simulink model "cantoni_combined_matrices_3pools_split"  (R2019b)
settings: Solver=FixedStepDiscrete  StartTime=0.0  StopTime=50  FixedStep=h  RelTol=1e-3
values from neighbouring files (symbols this model uses):
  comb_contr = ss(Ac, Bc, Cc, Dc, h)    [cantoni_LMI.m]
  comb_plant_disc = c2d(comb_plant_cont,h,'zoh')    [cantoni_LMI.m]
  ddelay = [4 2 4 4 6]    [distributed_workspace.mat]
undefined symbols (not defined in the file or in its folder): Pd, Wd
settings Model: Creator=Jacob  LastModifiedBy=bas
settings SFSimCC: CustomCodeUndefinedFunction=UseInterfaceOnly

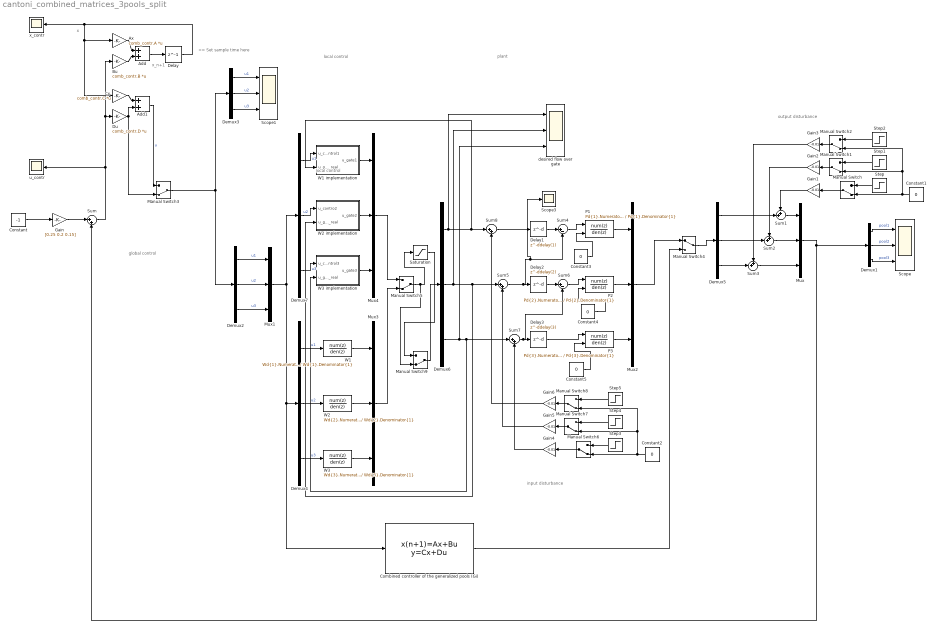
== system cantoni_combined_matrices_3pools_split ==
  note: input disturbance
  note: output disturbance
  note: local control
  note: <= Set sample time here
  note: plant
  note: local control
  note: global control
  note: x
  note: x_n+1
  Add : Sum
  Add1 : Sum
  Ax : Gain  Gain=comb_contr.A  Multiplication=Matrix(K*u)
  Bu : Gain  Gain=comb_contr.B  Multiplication=Matrix(K*u)
  Combined controller of the generalized pools (Gi) : DiscreteStateSpace  A=comb_plant_disc.A  B=comb_plant_disc.B  C=comb_plant_disc.C  D=comb_plant_disc.D  SampleTime=-1
  Constant : Constant  Value=-1
  Constant{1..2,4..5} (4 alike) : Constant  Value=0
  Constant3 : Constant  Value=0  SampleTime=-1
  Cx : Gain  Gain=comb_contr.C  Multiplication=Matrix(K*u)
  Delay : Delay  DelayLength=1  InitialCondition=[0;0;0;0;0;0;0;0;0;0;0;0;0;0;0]
  Delay1 : Delay  DelayLength=ddelay(1)
  Delay2 : Delay  DelayLength=ddelay(2)
  Delay3 : Delay  DelayLength=ddelay(3)
  Demux{1..7} (7 alike) : Demux  Outputs=3
  Du : Gain  Gain=comb_contr.D  Multiplication=Matrix(K*u)
  Gain : Gain  Gain=[0.25 0.2 0.15]
  Gain{1..6} (6 alike) : Gain  Gain=-0.01
  Manual Switch{,1..3,5..9} (9 alike) : ManualSwitch  CurrentSetting=0
  Manual Switch4 : ManualSwitch
  Mux{,1..4} (5 alike) : Mux  Inputs=3
  P1 : DiscreteTransferFcn  Numerator=Pd{1}.Numerator{1}  Denominator=Pd{1}.Denominator{1}  InitialStatesSource=Input port
      settings: InputPortMap=u0,p5
  P2 : DiscreteTransferFcn  Numerator=Pd{2}.Numerator{1}  Denominator=Pd{2}.Denominator{1}  InitialStatesSource=Input port
      settings: InputPortMap=u0,p5
  P3 : DiscreteTransferFcn  Numerator=Pd{3}.Numerator{1}  Denominator=Pd{3}.Denominator{1}  InitialStatesSource=Input port
      settings: InputPortMap=u0,p5
  Saturation : Saturate  UpperLimit=0.005  LowerLimit=-0.0001
  Scope : Scope  NumInputPorts=3
  Scope1 : Scope  NumInputPorts=3
  Scope3 : Scope
  Step{,1..5} (6 alike) : Step  Time=50  SampleTime=0
  Sum{,5,7..8} (4 alike) : Sum  Inputs=|++
  Sum1 : Sum  Inputs=++|
  Sum2 : Sum  Inputs=++|
  Sum3 : Sum  Inputs=++|
  Sum4 : Sum  Inputs=|+-
  Sum6 : Sum  Inputs=|+-
  W1 : DiscreteTransferFcn  Numerator=Wd{1}.Numerator{1}  Denominator=Wd{1}.Denominator{1}
  W1 implementation : Subsystem
  W2 : DiscreteTransferFcn  Numerator=Wd{2}.Numerator{1}  Denominator=Wd{2}.Denominator{1}
  W2 implementation : Subsystem
  W3 : DiscreteTransferFcn  Numerator=Wd{3}.Numerator{1}  Denominator=Wd{3}.Denominator{1}
  W3 implementation : Subsystem
  desired flow over gate : Scope  NumInputPorts=3
  u_contr : Scope
  x_contr : Scope
  wires:
  Sum/1 -> Du/1, Bu/1, u_contr/1
  Constant/1 -> Gain/1
  Gain/1 -> Sum/1
  Mux/1 -> Demux1/1, Sum/2
  Demux1/1 -> Scope/1  "pool1"
  Demux1/2 -> Scope/2  "pool2"
  Demux1/3 -> Scope/3  "pool3"
  Step/1 -> Manual Switch/1
  Sum1/1 -> Mux/1
  Sum2/1 -> Mux/2
  Gain2/1 -> Sum2/1
  Step1/1 -> Manual Switch1/1
  Gain1/1 -> Sum1/1
  Manual Switch/1 -> Gain1/1
  Constant1/1 -> Manual Switch1/2, Manual Switch2/2, Manual Switch/2
  Manual Switch1/1 -> Gain2/1
  Sum3/1 -> Mux/3
  Manual Switch2/1 -> Gain3/1
  Step2/1 -> Manual Switch2/1
  Gain3/1 -> Sum3/1
  Demux2/3 -> Mux1/3  "u3"
  Demux2/2 -> Mux1/2  "u2"
  Demux3/3 -> Scope1/3  "u3"
  Demux3/2 -> Scope1/2  "u2"
  Demux3/1 -> Scope1/1  "u1"
  Ax/1 -> Add/1
  Add/1 -> Delay/1
  Bu/1 -> Add/2
  Delay/1 -> x_contr/1, Cx/1, Ax/1
  Cx/1 -> Add1/1
  Du/1 -> Manual Switch3/2, Add1/2
  Add1/1 -> Manual Switch3/1  "u"
  Manual Switch3/1 -> Demux2/1, Demux3/1
  Demux2/1 -> Mux1/1  "u1"
  Demux5/1 -> Sum1/2
  Demux5/2 -> Sum2/2
  Demux5/3 -> Sum3/2
  Mux1/1 -> Combined controller of the generalized pools (Gi)/1, Demux4/1, Demux7/1
  Demux4/1 -> W1/1  "u1"
  Demux4/2 -> W2/1  "u2"
  Demux4/3 -> W3/1  "u3"
  Manual Switch4/1 -> Demux5/1
  P1/1 -> Mux2/1
  P2/1 -> Mux2/2
  P3/1 -> Mux2/3
  Mux2/1 -> Manual Switch4/1
  Combined controller of the generalized pools (Gi)/1 -> Manual Switch4/2
  Sum4/1 -> P1/1
  Sum6/1 -> P2/1
  Demux6/1 -> W1 implementation/2(u_gate1_real), Sum8/1, desired flow over gate/1
  Demux6/2 -> W2 implementation/2(u_gate2_real), Sum5/1, desired flow over gate/2
  Demux6/3 -> W3 implementation/2(u_gate3_real), Sum7/1, desired flow over gate/3
  Delay1/1 -> Sum4/1
  Delay2/1 -> Sum6/1
  Delay3/1 -> P3/1
  W1/1 -> Mux3/1
  W1 implementation/1(u_gate1) -> Mux4/1
  W2/1 -> Mux3/2
  W3/1 -> Mux3/3
  Mux3/1 -> Manual Switch5/2
  Demux7/1 -> W1 implementation/1(u_control1)  "u1"
  Mux4/1 -> Manual Switch5/1
  Demux7/2 -> W2 implementation/1(u_contro2)  "u2"
  W2 implementation/1(u_gate2) -> Mux4/2
  W3 implementation/1(u_gate3) -> Mux4/3
  Demux7/3 -> W3 implementation/1(u_control3)  "u3"
  Gain5/1 -> Sum5/2
  Gain4/1 -> Sum7/2
  Manual Switch8/1 -> Gain6/1
  Step5/1 -> Manual Switch8/1
  Gain6/1 -> Sum8/2
  Constant2/1 -> Manual Switch7/2, Manual Switch8/2, Manual Switch6/2
  Manual Switch7/1 -> Gain5/1
  Step3/1 -> Manual Switch6/1
  Manual Switch6/1 -> Gain4/1
  Step4/1 -> Manual Switch7/1
  Sum8/1 -> Delay1/1
  Sum5/1 -> Scope3/1, Sum4/2, Delay2/1
  Sum7/1 -> Sum6/2, Delay3/1
  Constant3/1 -> P1/2
  Saturation/1 -> Manual Switch9/1
  Constant4/1 -> P2/2
  Constant5/1 -> P3/2
  Manual Switch5/1 -> Manual Switch9/2, Saturation/1
  Manual Switch9/1 -> Demux6/1

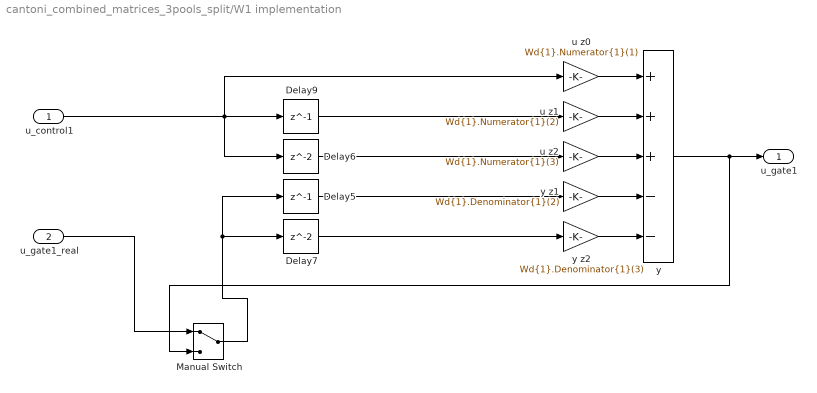
== system cantoni_combined_matrices_3pools_split/W1 implementation ==
  u_control1 : Inport
  u_gate1_real : Inport  Port=2
  Delay5 : Delay  DelayLength=1
  Delay6 : Delay
  Delay7 : Delay
  Delay9 : Delay  DelayLength=1
  Manual Switch : ManualSwitch
  u z0 : Gain  Gain=Wd{1}.Numerator{1}(1)
  u z1 : Gain  Gain=Wd{1}.Numerator{1}(2)
  u z2 : Gain  Gain=Wd{1}.Numerator{1}(3)
  y : Sum  Inputs=+++--
  y z1 : Gain  Gain=Wd{1}.Denominator{1}(2)
  y z2 : Gain  Gain=Wd{1}.Denominator{1}(3)
  u_gate1 : Outport
  wires:
  y z2/1 -> y/5
  Delay6/1 -> u z2/1
  y z1/1 -> y/4
  Delay7/1 -> y z2/1
  u z1/1 -> y/2
  u z2/1 -> y/3
  y/1 -> Manual Switch/2, u_gate1/1
  Delay5/1 -> y z1/1
  u_control1/1 -> Delay6/1, u z0/1, Delay9/1
  u z0/1 -> y/1
  Delay9/1 -> u z1/1
  Manual Switch/1 -> Delay5/1, Delay7/1
  u_gate1_real/1 -> Manual Switch/1

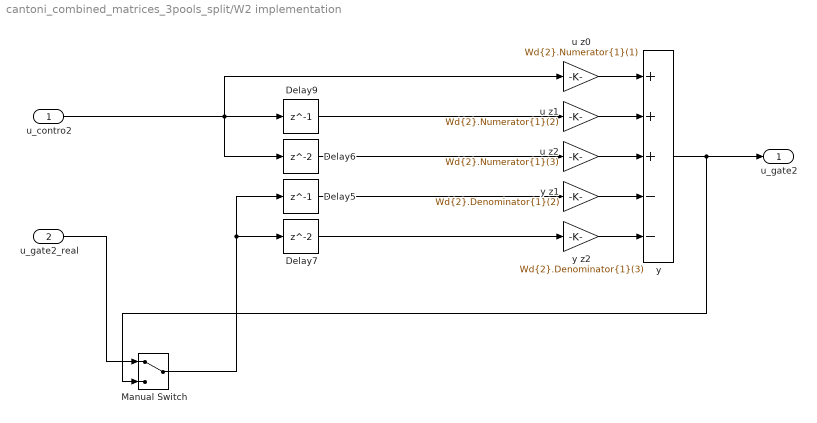
== system cantoni_combined_matrices_3pools_split/W2 implementation ==
  u_contro2 : Inport
  u_gate2_real : Inport  Port=2
  Delay5 : Delay  DelayLength=1
  Delay6 : Delay
  Delay7 : Delay
  Delay9 : Delay  DelayLength=1
  Manual Switch : ManualSwitch
  u z0 : Gain  Gain=Wd{2}.Numerator{1}(1)
  u z1 : Gain  Gain=Wd{2}.Numerator{1}(2)
  u z2 : Gain  Gain=Wd{2}.Numerator{1}(3)
  y : Sum  Inputs=+++--
  y z1 : Gain  Gain=Wd{2}.Denominator{1}(2)
  y z2 : Gain  Gain=Wd{2}.Denominator{1}(3)
  u_gate2 : Outport
  wires:
  y z2/1 -> y/5
  Delay6/1 -> u z2/1
  y z1/1 -> y/4
  Delay7/1 -> y z2/1
  u z1/1 -> y/2
  u z2/1 -> y/3
  y/1 -> Manual Switch/2, u_gate2/1
  Delay5/1 -> y z1/1
  u_contro2/1 -> Delay6/1, u z0/1, Delay9/1
  u z0/1 -> y/1
  Delay9/1 -> u z1/1
  Manual Switch/1 -> Delay5/1, Delay7/1
  u_gate2_real/1 -> Manual Switch/1

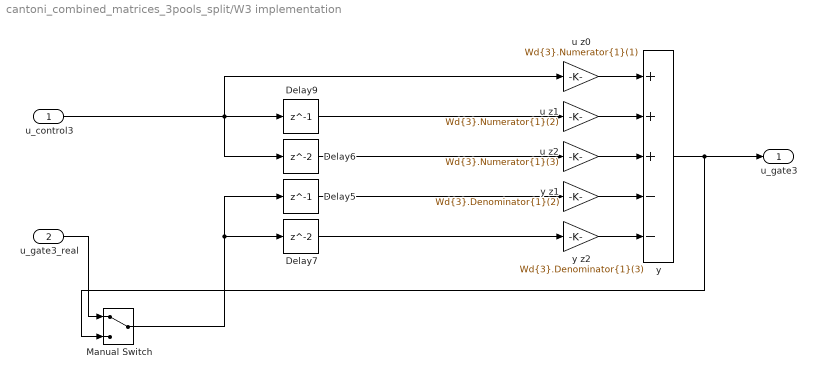
== system cantoni_combined_matrices_3pools_split/W3 implementation ==
  u_control3 : Inport
  u_gate3_real : Inport  Port=2
  Delay5 : Delay  DelayLength=1
  Delay6 : Delay
  Delay7 : Delay
  Delay9 : Delay  DelayLength=1
  Manual Switch : ManualSwitch
  u z0 : Gain  Gain=Wd{3}.Numerator{1}(1)
  u z1 : Gain  Gain=Wd{3}.Numerator{1}(2)
  u z2 : Gain  Gain=Wd{3}.Numerator{1}(3)
  y : Sum  Inputs=+++--
  y z1 : Gain  Gain=Wd{3}.Denominator{1}(2)
  y z2 : Gain  Gain=Wd{3}.Denominator{1}(3)
  u_gate3 : Outport
  wires:
  y z2/1 -> y/5
  Delay6/1 -> u z2/1
  y z1/1 -> y/4
  Delay7/1 -> y z2/1
  u z1/1 -> y/2
  u z2/1 -> y/3
  y/1 -> Manual Switch/2, u_gate3/1
  Delay5/1 -> y z1/1
  u_control3/1 -> Delay6/1, u z0/1, Delay9/1
  u z0/1 -> y/1
  Delay9/1 -> u z1/1
  Manual Switch/1 -> Delay5/1, Delay7/1
  u_gate3_real/1 -> Manual Switch/1
